simulink model "W2P1"  (R2020b)
settings: Solver=VariableStepAuto  StartTime=0.0  StopTime=10.0  RelTol=1e-3
settings Model: Creator=ASUS  LastModifiedBy=ASUS

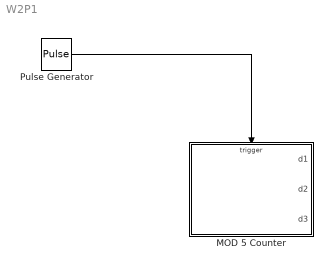
== system W2P1 ==
  MOD 5 Counter : Stateflow chart  TreatAsAtomicUnit=on
  Pulse Generator : DiscretePulseGenerator  PulseType=Time based  Period=0.01  PulseWidth=5  PhaseDelay=0.1
  wires:
  Pulse Generator/1 -> MOD 5 Counter/Trigger

== stateflow chart W2P1/MOD 5 Counter ==
  settings: executeAtInitialization=1
  state d2 [parallel]
    settings: executionOrder=2
    state one
      en:
      d2=1;
    state zero
      en:
      d2=0;
    state two
      en:
      d2=2;
    state four
      en:
      d2=4;
    state three
      en:
      d2=3;
    d2.zero -> d2.one : inc2
    d2.one -> d2.two : inc2
    (default) -> d2.zero
    d2.four -> d2.zero : inc2/{inc3}
    d2.two -> d2.three : inc2
    d2.three -> d2.four : inc2
  state d1 [parallel]
    settings: executionOrder=1
    state one
      en:
      d1=1;
    state zero
      en:
      d1=0;
    state two
      en:
      d1=2;
    state four
      en:
      d1=4;
    state three
      en:
      d1=3;
    d1.zero -> d1.one : inc1
    d1.one -> d1.two : inc1
    (default) -> d1.zero
    d1.four -> d1.zero : inc1/{inc2}
    d1.two -> d1.three : inc1
    d1.three -> d1.four : inc1
  state d3 [parallel]
    settings: executionOrder=3
    state one
      en:
      d3=1;
    state zero
      en:
      d3=0;
    state two
      en:
      d3=2;
    state four
      en:
      d3=4;
    state three1
      en:
      d3=3;
    d3.zero -> d3.one : inc3
    d3.one -> d3.two : inc3
    (default) -> d3.zero
    d3.four -> d3.zero : inc3
    d3.two -> three1 : inc3
    three1 -> d3.four : inc3
  data: d1 output size=1; d2 output size=1; d3 output size=1
  events: inc3 local FUNCTION_CALL_EVENT; inc2 local RISING_EDGE_EVENT; inc1 input RISING_EDGE_EVENT
